simulink model "PROBLEM3"  (R2020b)
settings: Solver=VariableStepAuto  StartTime=0.0  StopTime=100  RelTol=1e-3
undefined symbols (not defined in the file or in its folder): b, Kd, Ki, Kp, m
settings Model: Creator=ARPITA  LastModifiedBy=ARPITA

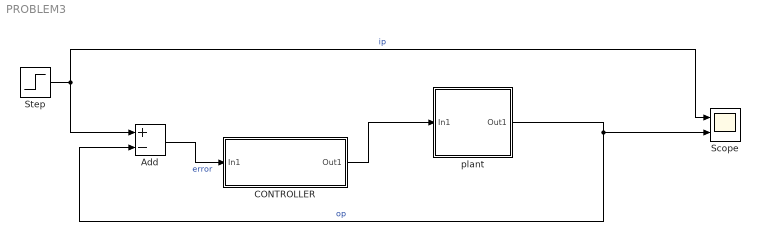
== system PROBLEM3 ==
  Add : Sum  Inputs=+-
  CONTROLLER : Subsystem
  Scope : Scope  NumInputPorts=2
  Step : Step  Time=0  Before=1  After=500  SampleTime=0
  plant : Subsystem
  wires:
  Step/1 -> Add/1, Scope/1  "ip"
  plant/1(Out1) -> Scope/2, Add/2  "op"
  CONTROLLER/1(Out1) -> plant/1(In1)
  Add/1 -> CONTROLLER/1(In1)  "error"

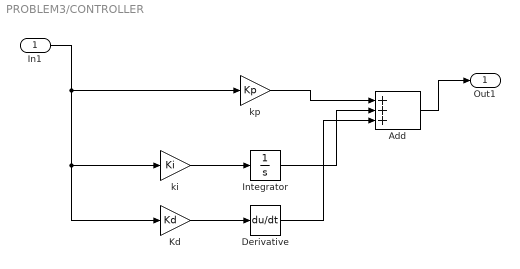
== system PROBLEM3/CONTROLLER ==
  In1 : Inport
  Add : Sum  Inputs=+++
  Derivative : Derivative
  Integrator : Integrator
  Kd : Gain  Gain=Kd
  ki : Gain  Gain=Ki
  kp : Gain  Gain=Kp
  Out1 : Outport
  wires:
  Derivative/1 -> Add/3
  kp/1 -> Add/1
  Kd/1 -> Derivative/1
  Integrator/1 -> Add/2
  ki/1 -> Integrator/1
  Add/1 -> Out1/1
  In1/1 -> Kd/1, ki/1, kp/1

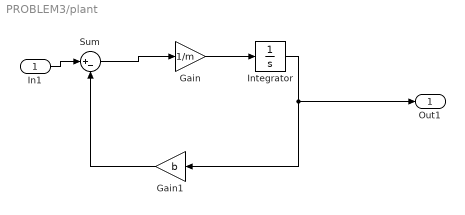
== system PROBLEM3/plant ==
  In1 : Inport
  Gain : Gain  Gain=1/m
  Gain1 : Gain  Gain=b
  Integrator : Integrator
  Sum : Sum  Inputs=|+-
  Out1 : Outport
  wires:
  Gain1/1 -> Sum/2
  Integrator/1 -> Out1/1, Gain1/1
  Gain/1 -> Integrator/1
  Sum/1 -> Gain/1
  In1/1 -> Sum/1
